simulink library "constT_XYZvarZ_Ramp_cl"  (R2018b)
settings: Solver=VariableStepAuto  StartTime=0.0  StopTime=10.0  RelTol=1e-3
settings Model: Creator=mcobb  LastModifiedBy=mcobb

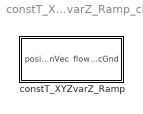
== system constT_XYZvarZ_Ramp_cl ==
  constT_XYZvarZ_Ramp : Subsystem  mask{flw=0}
      mask prompts: flw "env.constT_XYZvarZ_Ramp Object"
      settings: MinAlgLoopOccurrences=on

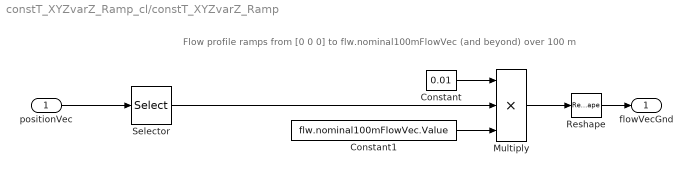
== system constT_XYZvarZ_Ramp_cl/constT_XYZvarZ_Ramp ==
  note: Flow profile ramps from [0 0 0] to flw.nominal100mFlowVec (and beyond) over 100 m
  positionVec : Inport
  Constant : Constant  Value=0.01
  Constant1 : Constant  Value=flw.nominal100mFlowVec.Value
  Multiply : Product  Inputs=3
  Reshape : Reshape  OutputDimensionality=Column vector (2-D)
  Selector : Selector  InputPortWidth=3  IndexOptions=Index vector (dialog)  Indices=3  OutputSizes=1
  flowVecGnd : Outport
  wires:
  positionVec/1 -> Selector/1
  Multiply/1 -> Reshape/1
  Reshape/1 -> flowVecGnd/1
  Constant/1 -> Multiply/1
  Constant1/1 -> Multiply/3
  Selector/1 -> Multiply/2
